simulink model "noise_response_basic"  (R2013a)
settings: Solver=ode45  StartTime=0.0  StopTime=10.0  RelTol=1e-3
settings Model: Creator=Colin  LastModifiedBy=Colin

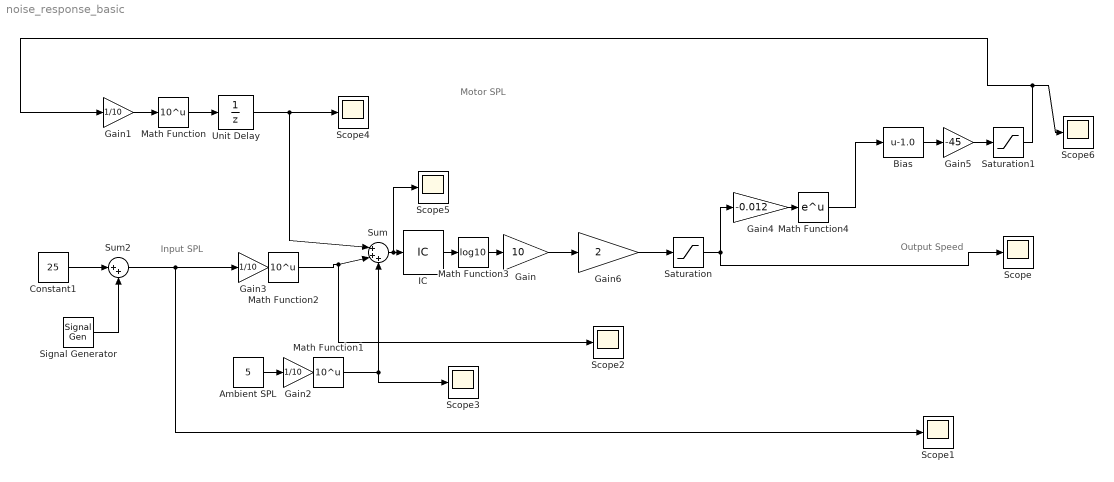
== system noise_response_basic ==
  note: Output Speed
  note: Input SPL
  note: Motor SPL
  Ambient SPL : Constant  Value=5
  Bias : Bias  Bias=-1.0
  Constant1 : Constant  Value=25
  Gain : Gain  Gain=10
  Gain1 : Gain  Gain=1/10
  Gain2 : Gain  Gain=1/10
  Gain3 : Gain  Gain=1/10
  Gain4 : Gain  Gain=-0.012
  Gain5 : Gain  Gain=-45
  Gain6 : Gain  Gain=2
  IC : InitialCondition  Value=30
  Math Function : Math  Operator=10^u  SaturateOnIntegerOverflow=on
  Math Function1 : Math  Operator=10^u  SaturateOnIntegerOverflow=on
  Math Function2 : Math  Operator=10^u  SaturateOnIntegerOverflow=on
  Math Function3 : Math  Operator=log10  SaturateOnIntegerOverflow=on
  Math Function4 : Math  SaturateOnIntegerOverflow=on
  Saturation : Saturate  UpperLimit=255  LowerLimit=0.5
  Saturation1 : Saturate  UpperLimit=60  LowerLimit=0.5
  Scope{,1..6} (7 alike) : Scope
      Scope2 settings: SaveName=ScopeData2
      Scope3 settings: SaveName=ScopeData3
      Scope4 settings: SaveName=ScopeData4
      Scope5 settings: SaveName=ScopeData5
      Scope6 settings: SaveName=ScopeData6
  Signal Generator : SignalGenerator  Amplitude=5  Frequency=0.4
  Sum : Sum  Inputs=|+++
  Sum2 : Sum  Inputs=|++
  Unit Delay : UnitDelay  SampleTime=-1
  wires:
  Gain2/1 -> Math Function1/1
  Gain3/1 -> Math Function2/1
  Gain1/1 -> Math Function/1
  Math Function3/1 -> Gain/1
  Ambient SPL/1 -> Gain2/1
  Gain4/1 -> Math Function4/1
  Math Function4/1 -> Bias/1
  Bias/1 -> Gain5/1
  Constant1/1 -> Sum2/1
  Signal Generator/1 -> Sum2/2
  Sum2/1 -> Scope1/1, Gain3/1
  Gain/1 -> Gain6/1
  Gain5/1 -> Saturation1/1
  Gain6/1 -> Saturation/1
  Sum/1 -> Scope5/1, IC/1
  Math Function1/1 -> Scope3/1, Sum/3
  Math Function2/1 -> Scope2/1, Sum/2
  IC/1 -> Math Function3/1
  Saturation/1 -> Scope/1, Gain4/1
  Math Function/1 -> Unit Delay/1
  Unit Delay/1 -> Sum/1, Scope4/1
  Saturation1/1 -> Gain1/1, Scope6/1
